simulink model "SystemComposerModel"  (R2022b)
settings: Solver=VariableStepAuto  StartTime=0.0  StopTime=10.0  RelTol=1e-3
(part 1 of 3)
settings Model: Creator=Daniel Sotelo  LastModifiedBy=teres
settings DebuggingCC: UnconnectedInputMsg=warning  UnconnectedOutputMsg=warning  UnconnectedLineMsg=warning
settings ModelReferenceCC: EnableRefExpFcnMdlSchedulingChecks=on
settings RTWCC: DLArmComputeVersion=19.05

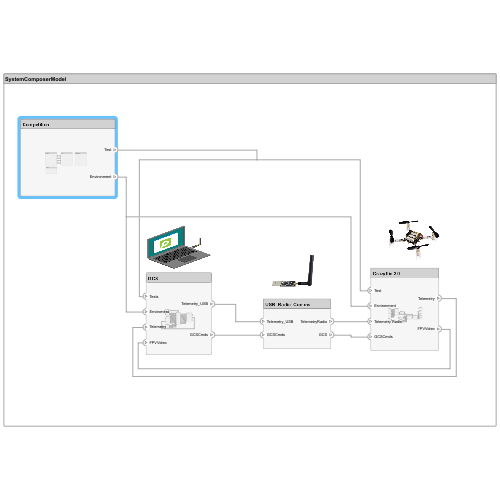
[thumbnail: Simulink's stored preview of the top-level diagram]
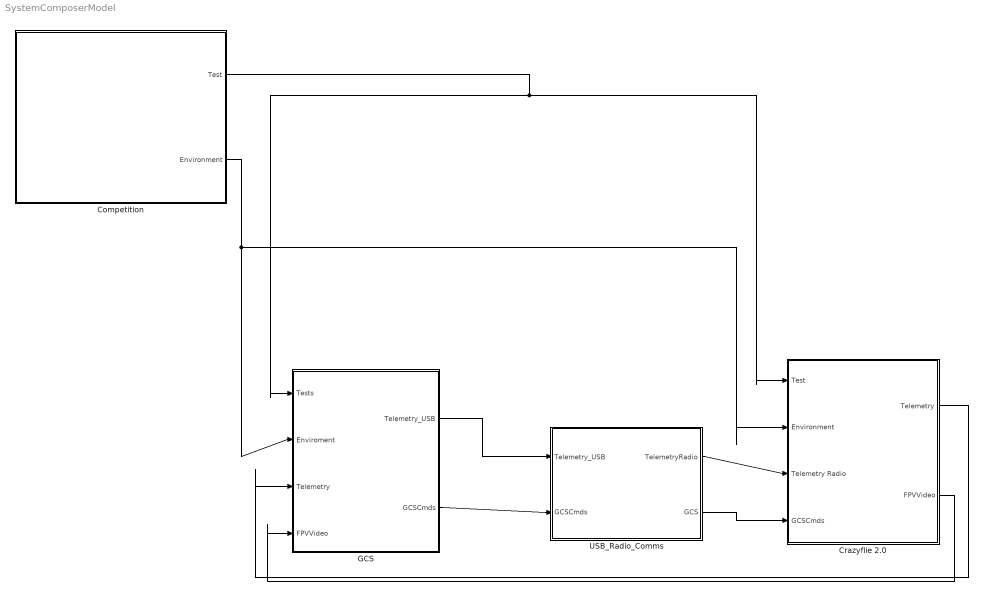
== system SystemComposerModel ==
  Competition : Subsystem
      settings: PortSchema="{\"entries\":[{\"content\":{\"headerSize\":26,\"margin\":15,\"minimumSpacing\":25,\"sides\":[{\"content\":{\"connectorIds\":[]},\"type\":\"ConnectorPlacement.EquallySpacedRectSide\",\"uuid\":\"fc8f1965-bed8-4a6e-9b63-950a000149c8\"},{\"content\":{\"connectorIds\":[\"Out1\",\"Out2\"],\"side\":\"RIGHT\"},\"type\":\"ConnectorPlacement.EquallySpacedRectSide\",\"uuid\":\"2c9d1f86-4f7d-4bcb-a56b-8c273be091e3\"},{\"content\":{\"connectorIds\":[],\"side\":\"TOP\"},\"type\":\"ConnectorPlacement.EquallySpacedRectSide\",\"uuid\":\"bf2fc06d-f400-4269-8d37-da038df58cba\"}]},\"type\":\"ConnectorPlacement.EquallySpacedConnector\",\"uuid\":\"4137853d-6a53-4ff1-a45c-0a11cac79d77\"}],\"packageUris\":[\"http://schema.mathworks.com/mf0/Connector/R2020b\"],\"version\":\"1.0\"}"
  Crazyflie 2.0 : Subsystem
      settings: PortSchema="{\"entries\":[{\"content\":{\"headerSize\":26,\"margin\":15,\"minimumSpacing\":25,\"sides\":[{\"content\":{\"connectorIds\":[\"In1\",\"In2\",\"In3\",\"In4\"]},\"type\":\"ConnectorPlacement.EquallySpacedRectSide\",\"uuid\":\"85361f62-a72a-43f7-8205-2bd06b4635eb\"},{\"content\":{\"connectorIds\":[\"Out1\",\"Out2\"],\"side\":\"RIGHT\"},\"type\":\"ConnectorPlacement.EquallySpacedRectSide\",\"uuid\":\"785bca03-4c5c-4ff5-9bb5-891ad5972055\"},{\"content\":{\"connectorIds\":[],\"side\":\"TOP\"},\"type\":\"ConnectorPlacement.EquallySpacedRectSide\",\"uuid\":\"4b8cfef5-38ba-456f-a828-b5cb7f165aef\"}]},\"type\":\"ConnectorPlacement.EquallySpacedConnector\",\"uuid\":\"8dffc657-0173-4421-b98e-59d56a4d09a6\"}],\"packageUris\":[\"http://schema.mathworks.com/mf0/Connector/R2020b\"],\"version\":\"1.0\"}"
  GCS : Subsystem
      settings: PortSchema="{\"entries\":[{\"content\":{\"headerSize\":26,\"margin\":15,\"minimumSpacing\":25,\"sides\":[{\"content\":{\"connectorIds\":[\"In1\",\"In2\",\"In3\",\"In4\"]},\"type\":\"ConnectorPlacement.EquallySpacedRectSide\",\"uuid\":\"b8d7d09c-e9ae-43de-8d46-f99ec2351e24\"},{\"content\":{\"connectorIds\":[\"Out1\",\"Out2\"],\"side\":\"RIGHT\"},\"type\":\"ConnectorPlacement.EquallySpacedRectSide\",\"uuid\":\"4693648e-b0a2-4db8-a983-4bee2f51d894\"},{\"content\":{\"connectorIds\":[],\"side\":\"TOP\"},\"type\":\"ConnectorPlacement.EquallySpacedRectSide\",\"uuid\":\"9f0e5fe3-4fa7-4597-a4df-94b2d5032736\"}]},\"type\":\"ConnectorPlacement.EquallySpacedConnector\",\"uuid\":\"297bf07a-4341-4423-8aed-0af6edbe7857\"}],\"packageUris\":[\"http://schema.mathworks.com/mf0/Connector/R2020b\"],\"version\":\"1.0\"}"
  USB_Radio_Comms : Subsystem
      settings: PortSchema="{\"entries\":[{\"content\":{\"headerSize\":26,\"margin\":15,\"minimumSpacing\":25,\"sides\":[{\"content\":{\"connectorIds\":[\"In1\",\"In2\"]},\"type\":\"ConnectorPlacement.EquallySpacedRectSide\",\"uuid\":\"3060b7dc-7094-4575-9bf7-25188df55435\"},{\"content\":{\"connectorIds\":[\"Out1\",\"Out2\"],\"side\":\"RIGHT\"},\"type\":\"ConnectorPlacement.EquallySpacedRectSide\",\"uuid\":\"b9a04f2f-3a87-4657-b996-549de6fa8c5c\"},{\"content\":{\"connectorIds\":[],\"side\":\"TOP\"},\"type\":\"ConnectorPlacement.EquallySpacedRectSide\",\"uuid\":\"d83a1232-3c8e-4ec4-b9bc-48e288d7909e\"}]},\"type\":\"ConnectorPlacement.EquallySpacedConnector\",\"uuid\":\"e5d04a2f-bf26-4a7e-a63c-4de52d3a604d\"}],\"packageUris\":[\"http://schema.mathworks.com/mf0/Connector/R2020b\"],\"version\":\"1.0\"}"
  wires:
  Crazyflie 2.0/1(Telemetry) -> GCS/3(Telemetry)
  Crazyflie 2.0/2(FPVVideo) -> GCS/4(FPVVideo)
  Competition/1(Test) -> GCS/1(Tests), Crazyflie 2.0/1(Test)
  Competition/2(Environment) -> Crazyflie 2.0/2(Environment), GCS/2(Enviroment)
  GCS/1(Telemetry_USB) -> USB_Radio_Comms/1(Telemetry_USB)
  GCS/2(GCSCmds) -> USB_Radio_Comms/2(GCSCmds)
  USB_Radio_Comms/1(TelemetryRadio) -> Crazyflie 2.0/3("Telemetry Radio ")
  USB_Radio_Comms/2(GCS) -> Crazyflie 2.0/4(GCSCmds)

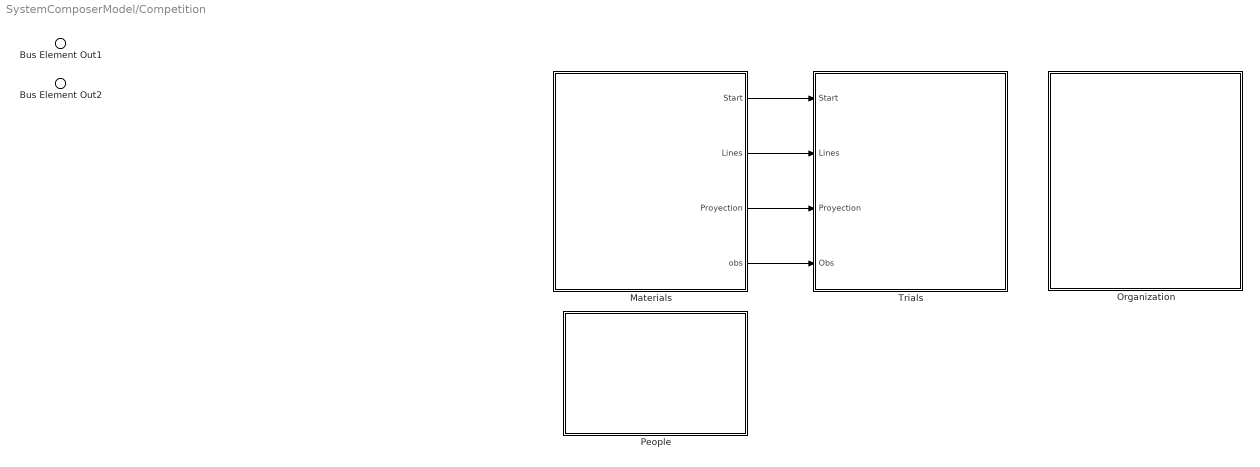
== system SystemComposerModel/Competition ==
  Materials : Subsystem
      settings: PortSchema="{\"entries\":[{\"content\":{\"headerSize\":26,\"margin\":15,\"minimumSpacing\":25,\"sides\":[{\"content\":{\"connectorIds\":[]},\"type\":\"ConnectorPlacement.EquallySpacedRectSide\",\"uuid\":\"036f86a6-46aa-44c7-aacf-5c5bf73f23a6\"},{\"content\":{\"connectorIds\":[\"Out1\",\"Out2\",\"Out3\",\"Out4\"],\"side\":\"RIGHT\"},\"type\":\"ConnectorPlacement.EquallySpacedRectSide\",\"uuid\":\"14d10c07-b9d4-4e69-9885-676f86520516\"},{\"content\":{\"connectorIds\":[],\"side\":\"TOP\"},\"type\":\"ConnectorPlacement.EquallySpacedRectSide\",\"uuid\":\"507b0a08-3f41-418e-b758-bf3c30bff976\"}]},\"type\":\"ConnectorPlacement.EquallySpacedConnector\",\"uuid\":\"3d035927-e5ab-4804-9878-aec4e1ed4314\"}],\"packageUris\":[\"http://schema.mathworks.com/mf0/Connector/R2020b\"],\"version\":\"1.0\"}"
  Organization : Subsystem
      settings: PortSchema="{\"entries\":[{\"content\":{\"headerSize\":26,\"margin\":15,\"minimumSpacing\":25,\"sides\":[{\"content\":{\"connectorIds\":[]},\"type\":\"ConnectorPlacement.EquallySpacedRectSide\",\"uuid\":\"036f86a6-46aa-44c7-aacf-5c5bf73f23a6\"},{\"content\":{\"connectorIds\":[],\"side\":\"RIGHT\"},\"type\":\"ConnectorPlacement.EquallySpacedRectSide\",\"uuid\":\"14d10c07-b9d4-4e69-9885-676f86520516\"},{\"content\":{\"connectorIds\":[],\"side\":\"TOP\"},\"type\":\"ConnectorPlacement.EquallySpacedRectSide\",\"uuid\":\"507b0a08-3f41-418e-b758-bf3c30bff976\"}]},\"type\":\"ConnectorPlacement.EquallySpacedConnector\",\"uuid\":\"3d035927-e5ab-4804-9878-aec4e1ed4314\"}],\"packageUris\":[\"http://schema.mathworks.com/mf0/Connector/R2020b\"],\"version\":\"1.0\"}"
  People : Subsystem
      settings: PortSchema="{\"entries\":[{\"content\":{\"headerSize\":26,\"margin\":15,\"minimumSpacing\":25,\"sides\":[{\"content\":{\"connectorIds\":[]},\"type\":\"ConnectorPlacement.EquallySpacedRectSide\",\"uuid\":\"036f86a6-46aa-44c7-aacf-5c5bf73f23a6\"},{\"content\":{\"connectorIds\":[],\"side\":\"RIGHT\"},\"type\":\"ConnectorPlacement.EquallySpacedRectSide\",\"uuid\":\"14d10c07-b9d4-4e69-9885-676f86520516\"},{\"content\":{\"connectorIds\":[],\"side\":\"TOP\"},\"type\":\"ConnectorPlacement.EquallySpacedRectSide\",\"uuid\":\"507b0a08-3f41-418e-b758-bf3c30bff976\"}]},\"type\":\"ConnectorPlacement.EquallySpacedConnector\",\"uuid\":\"3d035927-e5ab-4804-9878-aec4e1ed4314\"}],\"packageUris\":[\"http://schema.mathworks.com/mf0/Connector/R2020b\"],\"version\":\"1.0\"}"
  Trials : Subsystem
      settings: PortSchema="{\"entries\":[{\"content\":{\"headerSize\":26,\"margin\":15,\"minimumSpacing\":25,\"sides\":[{\"content\":{\"connectorIds\":[\"In1\",\"In2\",\"In3\",\"In4\"]},\"type\":\"ConnectorPlacement.EquallySpacedRectSide\",\"uuid\":\"036f86a6-46aa-44c7-aacf-5c5bf73f23a6\"},{\"content\":{\"connectorIds\":[],\"side\":\"RIGHT\"},\"type\":\"ConnectorPlacement.EquallySpacedRectSide\",\"uuid\":\"14d10c07-b9d4-4e69-9885-676f86520516\"},{\"content\":{\"connectorIds\":[],\"side\":\"TOP\"},\"type\":\"ConnectorPlacement.EquallySpacedRectSide\",\"uuid\":\"507b0a08-3f41-418e-b758-bf3c30bff976\"}]},\"type\":\"ConnectorPlacement.EquallySpacedConnector\",\"uuid\":\"3d035927-e5ab-4804-9878-aec4e1ed4314\"}],\"packageUris\":[\"http://schema.mathworks.com/mf0/Connector/R2020b\"],\"version\":\"1.0\"}"
  Bus Element Out1 : Outport  PortName=Test
  Bus Element Out2 : Outport  Port=2  PortName=Environment
  wires:
  Materials/2(Lines) -> Trials/2(Lines)
  Materials/3(Proyection) -> Trials/3(Proyection)
  Materials/4(obs) -> Trials/4(Obs)
  Materials/1(Start) -> Trials/1(Start)

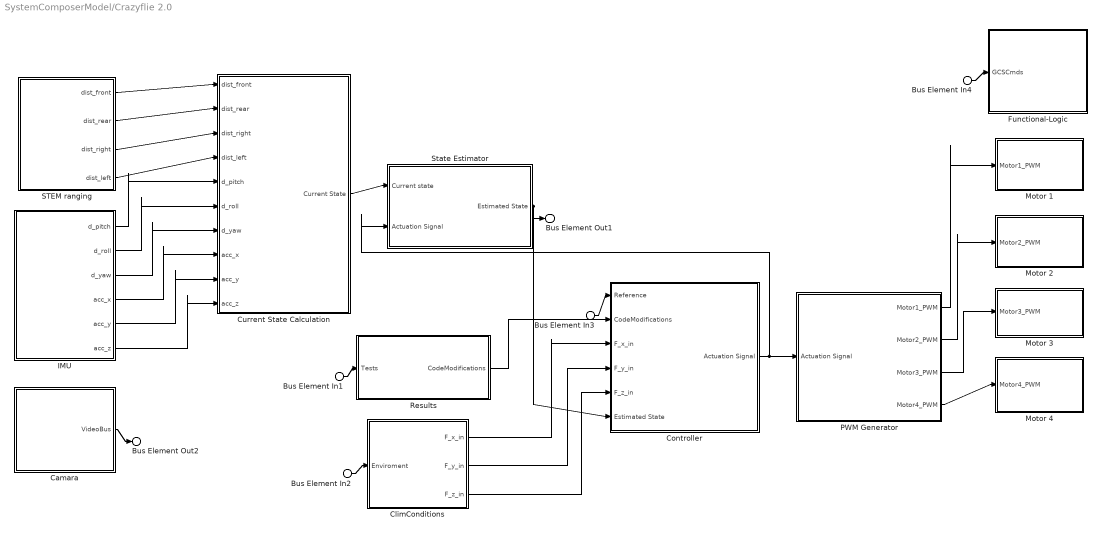
== system SystemComposerModel/Crazyflie 2.0 ==
  Bus Element In1 : Inport  PortName=Test
  Bus Element In2 : Inport  Port=2  PortName=Environment
  Bus Element In3 : Inport  Port=3  PortName=Telemetry Radio
  Bus Element In4 : Inport  Port=4  PortName=GCSCmds
  Camara : Subsystem
      settings: PortSchema="{\"entries\":[{\"content\":{\"headerSize\":26,\"margin\":15,\"minimumSpacing\":25,\"sides\":[{\"content\":{\"connectorIds\":[]},\"type\":\"ConnectorPlacement.EquallySpacedRectSide\",\"uuid\":\"85361f62-a72a-43f7-8205-2bd06b4635eb\"},{\"content\":{\"connectorIds\":[\"Out1\"],\"side\":\"RIGHT\"},\"type\":\"ConnectorPlacement.EquallySpacedRectSide\",\"uuid\":\"785bca03-4c5c-4ff5-9bb5-891ad5972055\"},{\"content\":{\"connectorIds\":[],\"side\":\"TOP\"},\"type\":\"ConnectorPlacement.EquallySpacedRectSide\",\"uuid\":\"4b8cfef5-38ba-456f-a828-b5cb7f165aef\"}]},\"type\":\"ConnectorPlacement.EquallySpacedConnector\",\"uuid\":\"8dffc657-0173-4421-b98e-59d56a4d09a6\"}],\"packageUris\":[\"http://schema.mathworks.com/mf0/Connector/R2020b\"],\"version\":\"1.0\"}"
  ClimConditions : Subsystem
      settings: PortSchema="{\"entries\":[{\"content\":{\"headerSize\":26,\"margin\":15,\"minimumSpacing\":25,\"sides\":[{\"content\":{\"connectorIds\":[\"In1\"]},\"type\":\"ConnectorPlacement.EquallySpacedRectSide\",\"uuid\":\"b8d7d09c-e9ae-43de-8d46-f99ec2351e24\"},{\"content\":{\"connectorIds\":[\"Out1\",\"Out2\",\"Out3\"],\"side\":\"RIGHT\"},\"type\":\"ConnectorPlacement.EquallySpacedRectSide\",\"uuid\":\"4693648e-b0a2-4db8-a983-4bee2f51d894\"},{\"content\":{\"connectorIds\":[],\"side\":\"TOP\"},\"type\":\"ConnectorPlacement.EquallySpacedRectSide\",\"uuid\":\"9f0e5fe3-4fa7-4597-a4df-94b2d5032736\"}]},\"type\":\"ConnectorPlacement.EquallySpacedConnector\",\"uuid\":\"297bf07a-4341-4423-8aed-0af6edbe7857\"}],\"packageUris\":[\"http://schema.mathworks.com/mf0/Connector/R2020b\"],\"version\":\"1.0\"}"
  Controller : Subsystem
      settings: PortSchema="{\"entries\":[{\"content\":{\"headerSize\":26,\"margin\":15,\"minimumSpacing\":25,\"sides\":[{\"content\":{\"connectorIds\":[\"In1\",\"In2\",\"In3\",\"In4\",\"In5\",\"In6\"]},\"type\":\"ConnectorPlacement.EquallySpacedRectSide\",\"uuid\":\"05353883-9549-4dc8-9a1c-5d1ae12c1484\"},{\"content\":{\"connectorIds\":[\"Out1\"],\"side\":\"RIGHT\"},\"type\":\"ConnectorPlacement.EquallySpacedRectSide\",\"uuid\":\"006c1520-45b5-4971-bef2-ea03737e2b23\"},{\"content\":{\"connectorIds\":[],\"side\":\"TOP\"},\"type\":\"ConnectorPlacement.EquallySpacedRectSide\",\"uuid\":\"e61f6cee-2c78-4df2-8cd1-114268c994e4\"}]},\"type\":\"ConnectorPlacement.EquallySpacedConnector\",\"uuid\":\"e2af53a5-fa78-4528-a754-d30d2cd5caf8\"}],\"packageUris\":[\"http://schema.mathworks.com/mf0/Connector/R2020b\"],\"version\":\"1.0\"}"
  Current State Calculation : Subsystem
      settings: PortSchema="{\"entries\":[{\"content\":{\"headerSize\":26,\"margin\":15,\"minimumSpacing\":25,\"sides\":[{\"content\":{\"connectorIds\":[\"In3\",\"In2\",\"In5\",\"In4\",\"In6\",\"In1\",\"In7\",\"In8\",\"In9\",\"In10\"]},\"type\":\"ConnectorPlacement.EquallySpacedRectSide\",\"uuid\":\"85361f62-a72a-43f7-8205-2bd06b4635eb\"},{\"content\":{\"connectorIds\":[\"Out1\"],\"side\":\"RIGHT\"},\"type\":\"ConnectorPlacement.EquallySpacedRectSide\",\"uuid\":\"785bca03-4c5c-4ff5-9bb5-891ad5972055\"},{\"content\":{\"connectorIds\":[],\"side\":\"TOP\"},\"type\":\"ConnectorPlacement.EquallySpacedRectSide\",\"uuid\":\"4b8cfef5-38ba-456f-a828-b5cb7f165aef\"},{\"content\":{\"connectorIds\":[],\"side\":\"BOTTOM\"},\"type\":\"ConnectorPlacement.EquallySpacedRectSide\",\"uuid\":\"ba702fc0-1fe6-457d-9dcb-728a63d76caf\"}]},\"type\":\"ConnectorPlacement.EquallySpacedConnector\",\"uuid\":\"8dffc657-0173-4421-b98e-59d56a4d09a6\"}],\"packageUris\":[\"http://schema.mathworks.com/mf0/Connector/R2020b\"],\"version\":\"1.0\"}"
  Functional-Logic : Subsystem
      settings: PortSchema="{\"entries\":[{\"content\":{\"headerSize\":26,\"margin\":15,\"minimumSpacing\":25,\"sides\":[{\"content\":{\"connectorIds\":[\"In1\"]},\"type\":\"ConnectorPlacement.EquallySpacedRectSide\",\"uuid\":\"85361f62-a72a-43f7-8205-2bd06b4635eb\"},{\"content\":{\"connectorIds\":[],\"side\":\"RIGHT\"},\"type\":\"ConnectorPlacement.EquallySpacedRectSide\",\"uuid\":\"785bca03-4c5c-4ff5-9bb5-891ad5972055\"},{\"content\":{\"connectorIds\":[],\"side\":\"TOP\"},\"type\":\"ConnectorPlacement.EquallySpacedRectSide\",\"uuid\":\"4b8cfef5-38ba-456f-a828-b5cb7f165aef\"}]},\"type\":\"ConnectorPlacement.EquallySpacedConnector\",\"uuid\":\"8dffc657-0173-4421-b98e-59d56a4d09a6\"}],\"packageUris\":[\"http://schema.mathworks.com/mf0/Connector/R2020b\"],\"version\":\"1.0\"}"
  IMU : Subsystem
      settings: PortSchema="{\"entries\":[{\"content\":{\"headerSize\":26,\"margin\":15,\"minimumSpacing\":25,\"sides\":[{\"content\":{\"connectorIds\":[]},\"type\":\"ConnectorPlacement.EquallySpacedRectSide\",\"uuid\":\"85361f62-a72a-43f7-8205-2bd06b4635eb\"},{\"content\":{\"connectorIds\":[\"Out1\",\"Out2\",\"Out3\",\"Out4\",\"Out5\",\"Out6\"],\"side\":\"RIGHT\"},\"type\":\"ConnectorPlacement.EquallySpacedRectSide\",\"uuid\":\"785bca03-4c5c-4ff5-9bb5-891ad5972055\"},{\"content\":{\"connectorIds\":[],\"side\":\"TOP\"},\"type\":\"ConnectorPlacement.EquallySpacedRectSide\",\"uuid\":\"4b8cfef5-38ba-456f-a828-b5cb7f165aef\"}]},\"type\":\"ConnectorPlacement.EquallySpacedConnector\",\"uuid\":\"8dffc657-0173-4421-b98e-59d56a4d09a6\"}],\"packageUris\":[\"http://schema.mathworks.com/mf0/Connector/R2020b\"],\"version\":\"1.0\"}"
  Motor 1 : Subsystem
      settings: PortSchema="{\"entries\":[{\"content\":{\"headerSize\":26,\"margin\":15,\"minimumSpacing\":25,\"sides\":[{\"content\":{\"connectorIds\":[\"In1\"]},\"type\":\"ConnectorPlacement.EquallySpacedRectSide\",\"uuid\":\"05353883-9549-4dc8-9a1c-5d1ae12c1484\"},{\"content\":{\"connectorIds\":[],\"side\":\"RIGHT\"},\"type\":\"ConnectorPlacement.EquallySpacedRectSide\",\"uuid\":\"006c1520-45b5-4971-bef2-ea03737e2b23\"},{\"content\":{\"connectorIds\":[],\"side\":\"TOP\"},\"type\":\"ConnectorPlacement.EquallySpacedRectSide\",\"uuid\":\"e61f6cee-2c78-4df2-8cd1-114268c994e4\"}]},\"type\":\"ConnectorPlacement.EquallySpacedConnector\",\"uuid\":\"e2af53a5-fa78-4528-a754-d30d2cd5caf8\"}],\"packageUris\":[\"http://schema.mathworks.com/mf0/Connector/R2020b\"],\"version\":\"1.0\"}"
  Motor 2 : Subsystem
      settings: PortSchema="{\"entries\":[{\"content\":{\"headerSize\":26,\"margin\":15,\"minimumSpacing\":25,\"sides\":[{\"content\":{\"connectorIds\":[\"In1\"]},\"type\":\"ConnectorPlacement.EquallySpacedRectSide\",\"uuid\":\"05353883-9549-4dc8-9a1c-5d1ae12c1484\"},{\"content\":{\"connectorIds\":[],\"side\":\"RIGHT\"},\"type\":\"ConnectorPlacement.EquallySpacedRectSide\",\"uuid\":\"006c1520-45b5-4971-bef2-ea03737e2b23\"},{\"content\":{\"connectorIds\":[],\"side\":\"TOP\"},\"type\":\"ConnectorPlacement.EquallySpacedRectSide\",\"uuid\":\"e61f6cee-2c78-4df2-8cd1-114268c994e4\"}]},\"type\":\"ConnectorPlacement.EquallySpacedConnector\",\"uuid\":\"e2af53a5-fa78-4528-a754-d30d2cd5caf8\"}],\"packageUris\":[\"http://schema.mathworks.com/mf0/Connector/R2020b\"],\"version\":\"1.0\"}"
  Motor 3 : Subsystem
      settings: PortSchema="{\"entries\":[{\"content\":{\"headerSize\":26,\"margin\":15,\"minimumSpacing\":25,\"sides\":[{\"content\":{\"connectorIds\":[\"In1\"]},\"type\":\"ConnectorPlacement.EquallySpacedRectSide\",\"uuid\":\"05353883-9549-4dc8-9a1c-5d1ae12c1484\"},{\"content\":{\"connectorIds\":[],\"side\":\"RIGHT\"},\"type\":\"ConnectorPlacement.EquallySpacedRectSide\",\"uuid\":\"006c1520-45b5-4971-bef2-ea03737e2b23\"},{\"content\":{\"connectorIds\":[],\"side\":\"TOP\"},\"type\":\"ConnectorPlacement.EquallySpacedRectSide\",\"uuid\":\"e61f6cee-2c78-4df2-8cd1-114268c994e4\"}]},\"type\":\"ConnectorPlacement.EquallySpacedConnector\",\"uuid\":\"e2af53a5-fa78-4528-a754-d30d2cd5caf8\"}],\"packageUris\":[\"http://schema.mathworks.com/mf0/Connector/R2020b\"],\"version\":\"1.0\"}"
  Motor 4 : Subsystem
      settings: PortSchema="{\"entries\":[{\"content\":{\"headerSize\":26,\"margin\":15,\"minimumSpacing\":25,\"sides\":[{\"content\":{\"connectorIds\":[\"In1\"]},\"type\":\"ConnectorPlacement.EquallySpacedRectSide\",\"uuid\":\"05353883-9549-4dc8-9a1c-5d1ae12c1484\"},{\"content\":{\"connectorIds\":[],\"side\":\"RIGHT\"},\"type\":\"ConnectorPlacement.EquallySpacedRectSide\",\"uuid\":\"006c1520-45b5-4971-bef2-ea03737e2b23\"},{\"content\":{\"connectorIds\":[],\"side\":\"TOP\"},\"type\":\"ConnectorPlacement.EquallySpacedRectSide\",\"uuid\":\"e61f6cee-2c78-4df2-8cd1-114268c994e4\"}]},\"type\":\"ConnectorPlacement.EquallySpacedConnector\",\"uuid\":\"e2af53a5-fa78-4528-a754-d30d2cd5caf8\"}],\"packageUris\":[\"http://schema.mathworks.com/mf0/Connector/R2020b\"],\"version\":\"1.0\"}"
  PWM Generator : Subsystem
      settings: PortSchema="{\"entries\":[{\"content\":{\"headerSize\":26,\"margin\":15,\"minimumSpacing\":25,\"sides\":[{\"content\":{\"connectorIds\":[\"In1\"]},\"type\":\"ConnectorPlacement.EquallySpacedRectSide\",\"uuid\":\"05353883-9549-4dc8-9a1c-5d1ae12c1484\"},{\"content\":{\"connectorIds\":[\"Out1\",\"Out2\",\"Out3\",\"Out4\"],\"side\":\"RIGHT\"},\"type\":\"ConnectorPlacement.EquallySpacedRectSide\",\"uuid\":\"006c1520-45b5-4971-bef2-ea03737e2b23\"},{\"content\":{\"connectorIds\":[],\"side\":\"TOP\"},\"type\":\"ConnectorPlacement.EquallySpacedRectSide\",\"uuid\":\"e61f6cee-2c78-4df2-8cd1-114268c994e4\"}]},\"type\":\"ConnectorPlacement.EquallySpacedConnector\",\"uuid\":\"e2af53a5-fa78-4528-a754-d30d2cd5caf8\"}],\"packageUris\":[\"http://schema.mathworks.com/mf0/Connector/R2020b\"],\"version\":\"1.0\"}"
  Results : Subsystem
      settings: PortSchema="{\"entries\":[{\"content\":{\"headerSize\":26,\"margin\":15,\"minimumSpacing\":25,\"sides\":[{\"content\":{\"connectorIds\":[\"In1\"]},\"type\":\"ConnectorPlacement.EquallySpacedRectSide\",\"uuid\":\"b8d7d09c-e9ae-43de-8d46-f99ec2351e24\"},{\"content\":{\"connectorIds\":[\"Out1\"],\"side\":\"RIGHT\"},\"type\":\"ConnectorPlacement.EquallySpacedRectSide\",\"uuid\":\"4693648e-b0a2-4db8-a983-4bee2f51d894\"},{\"content\":{\"connectorIds\":[],\"side\":\"TOP\"},\"type\":\"ConnectorPlacement.EquallySpacedRectSide\",\"uuid\":\"9f0e5fe3-4fa7-4597-a4df-94b2d5032736\"}]},\"type\":\"ConnectorPlacement.EquallySpacedConnector\",\"uuid\":\"297bf07a-4341-4423-8aed-0af6edbe7857\"}],\"packageUris\":[\"http://schema.mathworks.com/mf0/Connector/R2020b\"],\"version\":\"1.0\"}"
  STEM ranging : Subsystem
      settings: PortSchema="{\"entries\":[{\"content\":{\"headerSize\":26,\"margin\":15,\"minimumSpacing\":25,\"sides\":[{\"content\":{\"connectorIds\":[]},\"type\":\"ConnectorPlacement.EquallySpacedRectSide\",\"uuid\":\"85361f62-a72a-43f7-8205-2bd06b4635eb\"},{\"content\":{\"connectorIds\":[\"Out1\",\"Out2\",\"Out3\",\"Out4\"],\"side\":\"RIGHT\"},\"type\":\"ConnectorPlacement.EquallySpacedRectSide\",\"uuid\":\"785bca03-4c5c-4ff5-9bb5-891ad5972055\"},{\"content\":{\"connectorIds\":[],\"side\":\"TOP\"},\"type\":\"ConnectorPlacement.EquallySpacedRectSide\",\"uuid\":\"4b8cfef5-38ba-456f-a828-b5cb7f165aef\"}]},\"type\":\"ConnectorPlacement.EquallySpacedConnector\",\"uuid\":\"8dffc657-0173-4421-b98e-59d56a4d09a6\"}],\"packageUris\":[\"http://schema.mathworks.com/mf0/Connector/R2020b\"],\"version\":\"1.0\"}"
  State Estimator : Subsystem
      settings: PortSchema="{\"entries\":[{\"content\":{\"headerSize\":26,\"margin\":15,\"minimumSpacing\":25,\"sides\":[{\"content\":{\"connectorIds\":[\"In1\",\"In2\"]},\"type\":\"ConnectorPlacement.EquallySpacedRectSide\",\"uuid\":\"05353883-9549-4dc8-9a1c-5d1ae12c1484\"},{\"content\":{\"connectorIds\":[\"Out1\"],\"side\":\"RIGHT\"},\"type\":\"ConnectorPlacement.EquallySpacedRectSide\",\"uuid\":\"006c1520-45b5-4971-bef2-ea03737e2b23\"},{\"content\":{\"connectorIds\":[],\"side\":\"TOP\"},\"type\":\"ConnectorPlacement.EquallySpacedRectSide\",\"uuid\":\"e61f6cee-2c78-4df2-8cd1-114268c994e4\"}]},\"type\":\"ConnectorPlacement.EquallySpacedConnector\",\"uuid\":\"e2af53a5-fa78-4528-a754-d30d2cd5caf8\"}],\"packageUris\":[\"http://schema.mathworks.com/mf0/Connector/R2020b\"],\"version\":\"1.0\"}"
  Bus Element Out1 : Outport  PortName=Telemetry
  Bus Element Out2 : Outport  Port=2  PortName=FPVVideo
  wires:
  PWM Generator/3(Motor3_PWM) -> Motor 3/1(Motor3_PWM)
  STEM ranging/1(dist_front) -> Current State Calculation/3(dist_front)
  ClimConditions/2(F_y_in) -> Controller/4(F_y_in)
  STEM ranging/2(dist_rear) -> Current State Calculation/2(dist_rear)
  IMU/4(acc_x) -> Current State Calculation/8(acc_x)
  STEM ranging/4(dist_left) -> Current State Calculation/4(dist_left)
  STEM ranging/3(dist_right) -> Current State Calculation/5(dist_right)
  IMU/3(d_yaw) -> Current State Calculation/7(d_yaw)
  Results/1(CodeModifications) -> Controller/2(CodeModifications)
  IMU/2(d_roll) -> Current State Calculation/1(d_roll)
  IMU/1(d_pitch) -> Current State Calculation/6(d_pitch)
  IMU/5(acc_y) -> Current State Calculation/9(acc_y)
  IMU/6(acc_z) -> Current State Calculation/10(acc_z)
  Bus Element In4/1 -> Functional-Logic/1(GCSCmds)
  Camara/1(VideoBus) -> Bus Element Out2/1
  Current State Calculation/1(Current State) -> State Estimator/1(Current state)
  PWM Generator/2(Motor2_PWM) -> Motor 2/1(Motor2_PWM)
  Bus Element In2/1 -> ClimConditions/1(Enviroment)
  Bus Element In1/1 -> Results/1(Tests)
  PWM Generator/4(Motor4_PWM) -> Motor 4/1(Motor4_PWM)
  State Estimator/1(Estimated State) -> Controller/6(Estimated State), Bus Element Out1/1
  Controller/1(Actuation Signal) -> PWM Generator/1(Actuation Signal), State Estimator/2(Actuation Signal)
  Bus Element In3/1 -> Controller/1(Reference)
  ClimConditions/3(F_z_in) -> Controller/5(F_z_in)
  ClimConditions/1(F_x_in) -> Controller/3(F_x_in)
  PWM Generator/1(Motor1_PWM) -> Motor 1/1(Motor1_PWM)

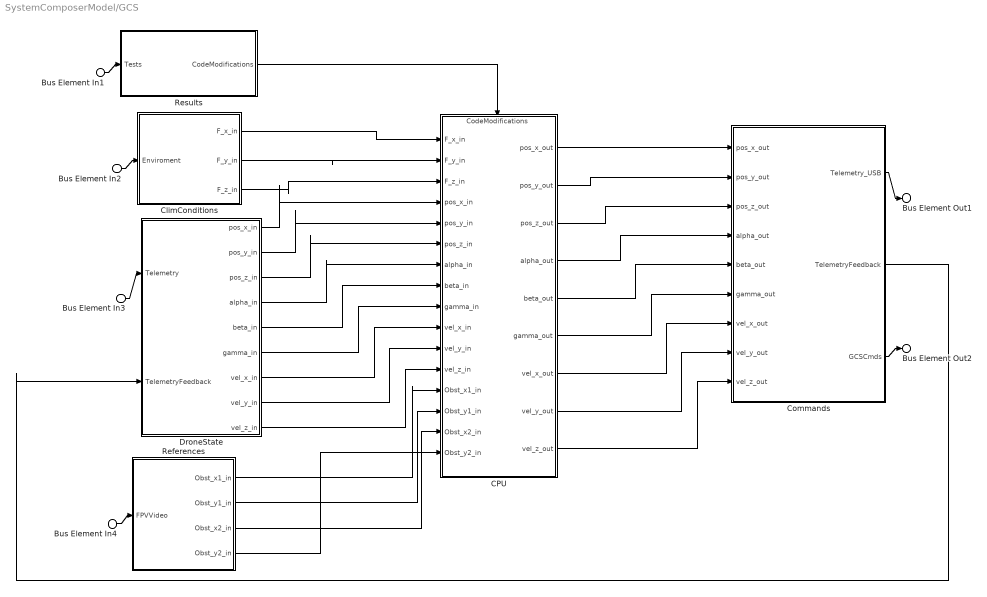
== system SystemComposerModel/GCS ==
  Bus Element In1 : Inport  PortName=Tests
  Bus Element In2 : Inport  Port=2  PortName=Enviroment
  Bus Element In3 : Inport  Port=3  PortName=Telemetry
  Bus Element In4 : Inport  Port=4  PortName=FPVVideo
  CPU : Subsystem
      settings: PortSchema="{\"entries\":[{\"content\":{\"headerSize\":26,\"margin\":15,\"minimumSpacing\":25,\"sides\":[{\"content\":{\"connectorIds\":[\"In2\",\"In3\",\"In4\",\"In5\",\"In6\",\"In7\",\"In8\",\"In9\",\"In10\",\"In11\",\"In12\",\"In13\",\"In14\",\"In15\",\"In16\",\"In17\"]},\"type\":\"ConnectorPlacement.EquallySpacedRectSide\",\"uuid\":\"b8d7d09c-e9ae-43de-8d46-f99ec2351e24\"},{\"content\":{\"connectorIds\":[\"Out1\",\"Out2\",\"Out3\",\"Out4\",\"Out5\",\"Out6\",\"Out7\",\"Out8\",\"Out9\"],\"side\":\"RIGHT\"},\"type\":\"ConnectorPlacement.EquallySpacedRectSide\",\"uuid\":\"4693648e-b0a2-4db8-a983-4bee2f51d894\"},{\"content\":{\"connectorIds\":[\"In1\"],\"side\":\"TOP\"},\"type\":\"ConnectorPlacement.EquallySpacedRectSide\",\"uuid\":\"9f0e5fe3-4fa7-4597-a4df-94b2d5032736\"}]},\"type\":\"ConnectorPlacement.EquallySpacedConnector\",\"uuid\":\"297bf07a-4341-4423-8aed-0af6edbe7857\"}],\"packageUris\":[\"http://schema.mathworks.com/mf0/Connector/R2020b\"],\"version\":\"1.0\"}"
  ClimConditions : Subsystem
      settings: PortSchema="{\"entries\":[{\"content\":{\"headerSize\":26,\"margin\":15,\"minimumSpacing\":25,\"sides\":[{\"content\":{\"connectorIds\":[\"In1\"]},\"type\":\"ConnectorPlacement.EquallySpacedRectSide\",\"uuid\":\"b8d7d09c-e9ae-43de-8d46-f99ec2351e24\"},{\"content\":{\"connectorIds\":[\"Out1\",\"Out2\",\"Out3\"],\"side\":\"RIGHT\"},\"type\":\"ConnectorPlacement.EquallySpacedRectSide\",\"uuid\":\"4693648e-b0a2-4db8-a983-4bee2f51d894\"},{\"content\":{\"connectorIds\":[],\"side\":\"TOP\"},\"type\":\"ConnectorPlacement.EquallySpacedRectSide\",\"uuid\":\"9f0e5fe3-4fa7-4597-a4df-94b2d5032736\"}]},\"type\":\"ConnectorPlacement.EquallySpacedConnector\",\"uuid\":\"297bf07a-4341-4423-8aed-0af6edbe7857\"}],\"packageUris\":[\"http://schema.mathworks.com/mf0/Connector/R2020b\"],\"version\":\"1.0\"}"
  Commands : Subsystem
      settings: PortSchema="{\"entries\":[{\"content\":{\"headerSize\":26,\"margin\":15,\"minimumSpacing\":25,\"sides\":[{\"content\":{\"connectorIds\":[\"In1\",\"In2\",\"In3\",\"In4\",\"In5\",\"In6\",\"In7\",\"In8\",\"In9\"]},\"type\":\"ConnectorPlacement.EquallySpacedRectSide\",\"uuid\":\"b8d7d09c-e9ae-43de-8d46-f99ec2351e24\"},{\"content\":{\"connectorIds\":[\"Out1\",\"Out2\",\"Out3\"],\"side\":\"RIGHT\"},\"type\":\"ConnectorPlacement.EquallySpacedRectSide\",\"uuid\":\"4693648e-b0a2-4db8-a983-4bee2f51d894\"},{\"content\":{\"connectorIds\":[],\"side\":\"TOP\"},\"type\":\"ConnectorPlacement.EquallySpacedRectSide\",\"uuid\":\"9f0e5fe3-4fa7-4597-a4df-94b2d5032736\"}]},\"type\":\"ConnectorPlacement.EquallySpacedConnector\",\"uuid\":\"297bf07a-4341-4423-8aed-0af6edbe7857\"}],\"packageUris\":[\"http://schema.mathworks.com/mf0/Connector/R2020b\"],\"version\":\"1.0\"}"
  DroneState : Subsystem
      settings: PortSchema="{\"entries\":[{\"content\":{\"headerSize\":26,\"margin\":15,\"minimumSpacing\":25,\"sides\":[{\"content\":{\"connectorIds\":[\"In1\",\"In2\"]},\"type\":\"ConnectorPlacement.EquallySpacedRectSide\",\"uuid\":\"b8d7d09c-e9ae-43de-8d46-f99ec2351e24\"},{\"content\":{\"connectorIds\":[\"Out1\",\"Out2\",\"Out3\",\"Out4\",\"Out5\",\"Out6\",\"Out7\",\"Out8\",\"Out9\"],\"side\":\"RIGHT\"},\"type\":\"ConnectorPlacement.EquallySpacedRectSide\",\"uuid\":\"4693648e-b0a2-4db8-a983-4bee2f51d894\"},{\"content\":{\"connectorIds\":[],\"side\":\"TOP\"},\"type\":\"ConnectorPlacement.EquallySpacedRectSide\",\"uuid\":\"9f0e5fe3-4fa7-4597-a4df-94b2d5032736\"}]},\"type\":\"ConnectorPlacement.EquallySpacedConnector\",\"uuid\":\"297bf07a-4341-4423-8aed-0af6edbe7857\"}],\"packageUris\":[\"http://schema.mathworks.com/mf0/Connector/R2020b\"],\"version\":\"1.0\"}"
  References : Subsystem
      settings: PortSchema="{\"entries\":[{\"content\":{\"headerSize\":26,\"margin\":15,\"minimumSpacing\":25,\"sides\":[{\"content\":{\"connectorIds\":[\"In1\"]},\"type\":\"ConnectorPlacement.EquallySpacedRectSide\",\"uuid\":\"b8d7d09c-e9ae-43de-8d46-f99ec2351e24\"},{\"content\":{\"connectorIds\":[\"Out1\",\"Out2\",\"Out3\",\"Out4\"],\"side\":\"RIGHT\"},\"type\":\"ConnectorPlacement.EquallySpacedRectSide\",\"uuid\":\"4693648e-b0a2-4db8-a983-4bee2f51d894\"},{\"content\":{\"connectorIds\":[],\"side\":\"TOP\"},\"type\":\"ConnectorPlacement.EquallySpacedRectSide\",\"uuid\":\"9f0e5fe3-4fa7-4597-a4df-94b2d5032736\"}]},\"type\":\"ConnectorPlacement.EquallySpacedConnector\",\"uuid\":\"297bf07a-4341-4423-8aed-0af6edbe7857\"}],\"packageUris\":[\"http://schema.mathworks.com/mf0/Connector/R2020b\"],\"version\":\"1.0\"}"
  Results : Subsystem
      settings: PortSchema="{\"entries\":[{\"content\":{\"headerSize\":26,\"margin\":15,\"minimumSpacing\":25,\"sides\":[{\"content\":{\"connectorIds\":[\"In1\"]},\"type\":\"ConnectorPlacement.EquallySpacedRectSide\",\"uuid\":\"b8d7d09c-e9ae-43de-8d46-f99ec2351e24\"},{\"content\":{\"connectorIds\":[\"Out1\"],\"side\":\"RIGHT\"},\"type\":\"ConnectorPlacement.EquallySpacedRectSide\",\"uuid\":\"4693648e-b0a2-4db8-a983-4bee2f51d894\"},{\"content\":{\"connectorIds\":[],\"side\":\"TOP\"},\"type\":\"ConnectorPlacement.EquallySpacedRectSide\",\"uuid\":\"9f0e5fe3-4fa7-4597-a4df-94b2d5032736\"}]},\"type\":\"ConnectorPlacement.EquallySpacedConnector\",\"uuid\":\"297bf07a-4341-4423-8aed-0af6edbe7857\"}],\"packageUris\":[\"http://schema.mathworks.com/mf0/Connector/R2020b\"],\"version\":\"1.0\"}"
  Bus Element Out1 : Outport  PortName=Telemetry_USB
  Bus Element Out2 : Outport  Port=2  PortName=GCSCmds
  wires:
  Bus Element In3/1 -> DroneState/1(Telemetry)
  Bus Element In4/1 -> References/1(FPVVideo)
  DroneState/1(pos_x_in) -> CPU/5(pos_x_in)
  DroneState/2(pos_y_in) -> CPU/6(pos_y_in)
  DroneState/3(pos_z_in) -> CPU/7(pos_z_in)
  DroneState/4(alpha_in) -> CPU/8(alpha_in)
  DroneState/5(beta_in) -> CPU/9(beta_in)
  DroneState/6(gamma_in) -> CPU/10(gamma_in)
  DroneState/7(vel_x_in) -> CPU/11(vel_x_in)
  DroneState/8(vel_y_in) -> CPU/12(vel_y_in)
  DroneState/9(vel_z_in) -> CPU/13(vel_z_in)
  References/1(Obst_x1_in) -> CPU/14(Obst_x1_in)
  References/2(Obst_y1_in) -> CPU/15(Obst_y1_in)
  References/3(Obst_x2_in) -> CPU/16(Obst_x2_in)
  References/4(Obst_y2_in) -> CPU/17(Obst_y2_in)
  Bus Element In2/1 -> ClimConditions/1(Enviroment)
  Bus Element In1/1 -> Results/1(Tests)
  ClimConditions/1(F_x_in) -> CPU/2(F_x_in)
  ClimConditions/2(F_y_in) -> CPU/3(F_y_in)
  ClimConditions/3(F_z_in) -> CPU/4(F_z_in)
  Results/1(CodeModifications) -> CPU/1(CodeModifications)
  CPU/1(pos_x_out) -> Commands/1(pos_x_out)
  CPU/2(pos_y_out) -> Commands/2(pos_y_out)
  CPU/3(pos_z_out) -> Commands/3(pos_z_out)
  CPU/4(alpha_out) -> Commands/4(alpha_out)
  CPU/5(beta_out) -> Commands/5(beta_out)
  CPU/6(gamma_out) -> Commands/6(gamma_out)
  CPU/7(vel_x_out) -> Commands/7(vel_x_out)
  CPU/8(vel_y_out) -> Commands/8(vel_y_out)
  CPU/9(vel_z_out) -> Commands/9(vel_z_out)
  Commands/3(GCSCmds) -> Bus Element Out2/1
  Commands/1(Telemetry_USB) -> Bus Element Out1/1
  Commands/2(TelemetryFeedback) -> DroneState/2(TelemetryFeedback)

== system SystemComposerModel/USB_Radio_Comms ==
  Bus Element In1 : Inport  PortName=Telemetry_USB
  Bus Element In2 : Inport  Port=2  PortName=GCSCmds
  Bus Element Out1 : Outport  PortName=TelemetryRadio
  Bus Element Out2 : Outport  Port=2  PortName=GCS

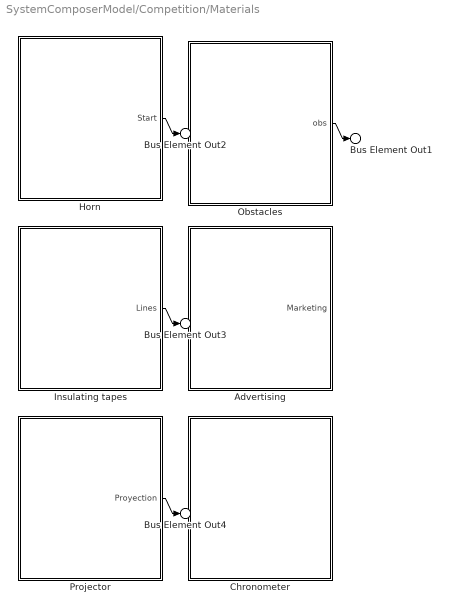
== system SystemComposerModel/Competition/Materials ==
  Advertising : Subsystem
      settings: PortSchema="{\"entries\":[{\"content\":{\"headerSize\":26,\"margin\":15,\"minimumSpacing\":25,\"sides\":[{\"content\":{\"connectorIds\":[]},\"type\":\"ConnectorPlacement.EquallySpacedRectSide\",\"uuid\":\"036f86a6-46aa-44c7-aacf-5c5bf73f23a6\"},{\"content\":{\"connectorIds\":[\"Out1\"],\"side\":\"RIGHT\"},\"type\":\"ConnectorPlacement.EquallySpacedRectSide\",\"uuid\":\"14d10c07-b9d4-4e69-9885-676f86520516\"},{\"content\":{\"connectorIds\":[],\"side\":\"TOP\"},\"type\":\"ConnectorPlacement.EquallySpacedRectSide\",\"uuid\":\"507b0a08-3f41-418e-b758-bf3c30bff976\"}]},\"type\":\"ConnectorPlacement.EquallySpacedConnector\",\"uuid\":\"3d035927-e5ab-4804-9878-aec4e1ed4314\"}],\"packageUris\":[\"http://schema.mathworks.com/mf0/Connector/R2020b\"],\"version\":\"1.0\"}"
  Chronometer : Subsystem  Description=|
      | Stopwatch needed to measure the time taken by the drone in the following tests:
      | 1. Speed test
      | 2. Tracking test
      | 3. Predefined obstacle test
      | 4. Random obstacle test
      | 5. Freestyle test
      | It will be sufficient to use the timer application included in the cell phones.
      settings: PortSchema="{\"entries\":[{\"content\":{\"headerSize\":26,\"margin\":15,\"minimumSpacing\":25,\"sides\":[{\"content\":{\"connectorIds\":[]},\"type\":\"ConnectorPlacement.EquallySpacedRectSide\",\"uuid\":\"036f86a6-46aa-44c7-aacf-5c5bf73f23a6\"},{\"content\":{\"connectorIds\":[],\"side\":\"RIGHT\"},\"type\":\"ConnectorPlacement.EquallySpacedRectSide\",\"uuid\":\"14d10c07-b9d4-4e69-9885-676f86520516\"},{\"content\":{\"connectorIds\":[],\"side\":\"TOP\"},\"type\":\"ConnectorPlacement.EquallySpacedRectSide\",\"uuid\":\"507b0a08-3f41-418e-b758-bf3c30bff976\"}]},\"type\":\"ConnectorPlacement.EquallySpacedConnector\",\"uuid\":\"3d035927-e5ab-4804-9878-aec4e1ed4314\"}],\"packageUris\":[\"http://schema.mathworks.com/mf0/Connector/R2020b\"],\"version\":\"1.0\"}"
  Horn : Subsystem  Description=|
      | Sound to mark the start of each test, in particular:
      | 1. Speed test
      | 2. Tracking test
      | 3. Predefined obstacle test
      | 4. Random obstacle test
      | 5. Freestyle test
      settings: PortSchema="{\"entries\":[{\"content\":{\"headerSize\":26,\"margin\":15,\"minimumSpacing\":25,\"sides\":[{\"content\":{\"connectorIds\":[]},\"type\":\"ConnectorPlacement.EquallySpacedRectSide\",\"uuid\":\"036f86a6-46aa-44c7-aacf-5c5bf73f23a6\"},{\"content\":{\"connectorIds\":[\"Out1\"],\"side\":\"RIGHT\"},\"type\":\"ConnectorPlacement.EquallySpacedRectSide\",\"uuid\":\"14d10c07-b9d4-4e69-9885-676f86520516\"},{\"content\":{\"connectorIds\":[],\"side\":\"TOP\"},\"type\":\"ConnectorPlacement.EquallySpacedRectSide\",\"uuid\":\"507b0a08-3f41-418e-b758-bf3c30bff976\"}]},\"type\":\"ConnectorPlacement.EquallySpacedConnector\",\"uuid\":\"3d035927-e5ab-4804-9878-aec4e1ed4314\"}],\"packageUris\":[\"http://schema.mathworks.com/mf0/Connector/R2020b\"],\"version\":\"1.0\"}"
  Insulating tapes : Subsystem  Description=|
      | Colored tape to delimit the course of each race, in particular:
      | 1. speed test: start and finish line (black) 
      | 2. Target test: marking on the ground the point from which the drone will take off (black).
      | 3. Trackline test: marking of the course (black color approx. 38mm thick, black color approx. 10mm thick, red color approx. 20mm thick), finish line (blue color).
      | 4. Predefined obstacle test: start and finish line.
      | 5. Random obstacle test: start and finish line.
      | 
      | For the above requirements, the following must be purchased:
      | 1 black tape approx. 38mm
      | 1 black tape approx. 10mm
      | 1 red tape approx. 20mm
      | 1 blue tape
      settings: PortSchema="{\"entries\":[{\"content\":{\"headerSize\":26,\"margin\":15,\"minimumSpacing\":25,\"sides\":[{\"content\":{\"connectorIds\":[]},\"type\":\"ConnectorPlacement.EquallySpacedRectSide\",\"uuid\":\"036f86a6-46aa-44c7-aacf-5c5bf73f23a6\"},{\"content\":{\"connectorIds\":[\"Out1\"],\"side\":\"RIGHT\"},\"type\":\"ConnectorPlacement.EquallySpacedRectSide\",\"uuid\":\"14d10c07-b9d4-4e69-9885-676f86520516\"},{\"content\":{\"connectorIds\":[],\"side\":\"TOP\"},\"type\":\"ConnectorPlacement.EquallySpacedRectSide\",\"uuid\":\"507b0a08-3f41-418e-b758-bf3c30bff976\"}]},\"type\":\"ConnectorPlacement.EquallySpacedConnector\",\"uuid\":\"3d035927-e5ab-4804-9878-aec4e1ed4314\"}],\"packageUris\":[\"http://schema.mathworks.com/mf0/Connector/R2020b\"],\"version\":\"1.0\"}"
  Obstacles : Subsystem
      settings: PortSchema="{\"entries\":[{\"content\":{\"headerSize\":26,\"margin\":15,\"minimumSpacing\":25,\"sides\":[{\"content\":{\"connectorIds\":[]},\"type\":\"ConnectorPlacement.EquallySpacedRectSide\",\"uuid\":\"036f86a6-46aa-44c7-aacf-5c5bf73f23a6\"},{\"content\":{\"connectorIds\":[\"Out1\"],\"side\":\"RIGHT\"},\"type\":\"ConnectorPlacement.EquallySpacedRectSide\",\"uuid\":\"14d10c07-b9d4-4e69-9885-676f86520516\"},{\"content\":{\"connectorIds\":[],\"side\":\"TOP\"},\"type\":\"ConnectorPlacement.EquallySpacedRectSide\",\"uuid\":\"507b0a08-3f41-418e-b758-bf3c30bff976\"}]},\"type\":\"ConnectorPlacement.EquallySpacedConnector\",\"uuid\":\"3d035927-e5ab-4804-9878-aec4e1ed4314\"}],\"packageUris\":[\"http://schema.mathworks.com/mf0/Connector/R2020b\"],\"version\":\"1.0\"}"
  Projector : Subsystem  Description=Projector connected to a computer, capable of projecting on a smooth wall everything necessary to carry out the target test.
      settings: PortSchema="{\"entries\":[{\"content\":{\"headerSize\":26,\"margin\":15,\"minimumSpacing\":25,\"sides\":[{\"content\":{\"connectorIds\":[]},\"type\":\"ConnectorPlacement.EquallySpacedRectSide\",\"uuid\":\"036f86a6-46aa-44c7-aacf-5c5bf73f23a6\"},{\"content\":{\"connectorIds\":[\"Out1\"],\"side\":\"RIGHT\"},\"type\":\"ConnectorPlacement.EquallySpacedRectSide\",\"uuid\":\"14d10c07-b9d4-4e69-9885-676f86520516\"},{\"content\":{\"connectorIds\":[],\"side\":\"TOP\"},\"type\":\"ConnectorPlacement.EquallySpacedRectSide\",\"uuid\":\"507b0a08-3f41-418e-b758-bf3c30bff976\"}]},\"type\":\"ConnectorPlacement.EquallySpacedConnector\",\"uuid\":\"3d035927-e5ab-4804-9878-aec4e1ed4314\"}],\"packageUris\":[\"http://schema.mathworks.com/mf0/Connector/R2020b\"],\"version\":\"1.0\"}"
  Bus Element Out2 : Outport  PortName=Start
  Bus Element Out3 : Outport  Port=2  PortName=Lines
  Bus Element Out4 : Outport  Port=3  PortName=Proyection
  Bus Element Out1 : Outport  Port=4  PortName=obs
  wires:
  Obstacles/1(obs) -> Bus Element Out1/1
  Horn/1(Start) -> Bus Element Out2/1
  Insulating tapes/1(Lines) -> Bus Element Out3/1
  Projector/1(Proyection) -> Bus Element Out4/1

== system SystemComposerModel/Competition/Organization ==
  Before the competition : Subsystem
      settings: PortSchema="{\"entries\":[{\"content\":{\"headerSize\":26,\"margin\":15,\"minimumSpacing\":25,\"sides\":[{\"content\":{\"connectorIds\":[]},\"type\":\"ConnectorPlacement.EquallySpacedRectSide\",\"uuid\":\"d34c32ef-3d27-469b-8a35-abebe5333993\"},{\"content\":{\"connectorIds\":[],\"side\":\"RIGHT\"},\"type\":\"ConnectorPlacement.EquallySpacedRectSide\",\"uuid\":\"0a2917af-f234-4cdf-997c-680a118988b7\"},{\"content\":{\"connectorIds\":[],\"side\":\"TOP\"},\"type\":\"ConnectorPlacement.EquallySpacedRectSide\",\"uuid\":\"dcac7d54-9fff-4582-ba14-08bcbac36cd8\"}]},\"type\":\"ConnectorPlacement.EquallySpacedConnector\",\"uuid\":\"84591ee6-ffcc-49ff-97f7-997353b331d9\"}],\"packageUris\":[\"http://schema.mathworks.com/mf0/Connector/R2020b\"],\"version\":\"1.0\"}"
  During the competition : Subsystem
      settings: PortSchema="{\"entries\":[{\"content\":{\"headerSize\":26,\"margin\":15,\"minimumSpacing\":25,\"sides\":[{\"content\":{\"connectorIds\":[]},\"type\":\"ConnectorPlacement.EquallySpacedRectSide\",\"uuid\":\"d34c32ef-3d27-469b-8a35-abebe5333993\"},{\"content\":{\"connectorIds\":[],\"side\":\"RIGHT\"},\"type\":\"ConnectorPlacement.EquallySpacedRectSide\",\"uuid\":\"0a2917af-f234-4cdf-997c-680a118988b7\"},{\"content\":{\"connectorIds\":[],\"side\":\"TOP\"},\"type\":\"ConnectorPlacement.EquallySpacedRectSide\",\"uuid\":\"dcac7d54-9fff-4582-ba14-08bcbac36cd8\"}]},\"type\":\"ConnectorPlacement.EquallySpacedConnector\",\"uuid\":\"84591ee6-ffcc-49ff-97f7-997353b331d9\"}],\"packageUris\":[\"http://schema.mathworks.com/mf0/Connector/R2020b\"],\"version\":\"1.0\"}"

== system SystemComposerModel/Competition/People ==
  Audience : Subsystem
      settings: PortSchema="{\"entries\":[{\"content\":{\"headerSize\":26,\"margin\":15,\"minimumSpacing\":25,\"sides\":[{\"content\":{\"connectorIds\":[]},\"type\":\"ConnectorPlacement.EquallySpacedRectSide\",\"uuid\":\"036f86a6-46aa-44c7-aacf-5c5bf73f23a6\"},{\"content\":{\"connectorIds\":[],\"side\":\"RIGHT\"},\"type\":\"ConnectorPlacement.EquallySpacedRectSide\",\"uuid\":\"14d10c07-b9d4-4e69-9885-676f86520516\"},{\"content\":{\"connectorIds\":[],\"side\":\"TOP\"},\"type\":\"ConnectorPlacement.EquallySpacedRectSide\",\"uuid\":\"507b0a08-3f41-418e-b758-bf3c30bff976\"}]},\"type\":\"ConnectorPlacement.EquallySpacedConnector\",\"uuid\":\"3d035927-e5ab-4804-9878-aec4e1ed4314\"}],\"packageUris\":[\"http://schema.mathworks.com/mf0/Connector/R2020b\"],\"version\":\"1.0\"}"
  Observers : Subsystem
      settings: PortSchema="{\"entries\":[{\"content\":{\"headerSize\":26,\"margin\":15,\"minimumSpacing\":25,\"sides\":[{\"content\":{\"connectorIds\":[]},\"type\":\"ConnectorPlacement.EquallySpacedRectSide\",\"uuid\":\"036f86a6-46aa-44c7-aacf-5c5bf73f23a6\"},{\"content\":{\"connectorIds\":[],\"side\":\"RIGHT\"},\"type\":\"ConnectorPlacement.EquallySpacedRectSide\",\"uuid\":\"14d10c07-b9d4-4e69-9885-676f86520516\"},{\"content\":{\"connectorIds\":[],\"side\":\"TOP\"},\"type\":\"ConnectorPlacement.EquallySpacedRectSide\",\"uuid\":\"507b0a08-3f41-418e-b758-bf3c30bff976\"}]},\"type\":\"ConnectorPlacement.EquallySpacedConnector\",\"uuid\":\"3d035927-e5ab-4804-9878-aec4e1ed4314\"}],\"packageUris\":[\"http://schema.mathworks.com/mf0/Connector/R2020b\"],\"version\":\"1.0\"}"
  Participants : Subsystem
      settings: PortSchema="{\"entries\":[{\"content\":{\"headerSize\":26,\"margin\":15,\"minimumSpacing\":25,\"sides\":[{\"content\":{\"connectorIds\":[]},\"type\":\"ConnectorPlacement.EquallySpacedRectSide\",\"uuid\":\"036f86a6-46aa-44c7-aacf-5c5bf73f23a6\"},{\"content\":{\"connectorIds\":[],\"side\":\"RIGHT\"},\"type\":\"ConnectorPlacement.EquallySpacedRectSide\",\"uuid\":\"14d10c07-b9d4-4e69-9885-676f86520516\"},{\"content\":{\"connectorIds\":[],\"side\":\"TOP\"},\"type\":\"ConnectorPlacement.EquallySpacedRectSide\",\"uuid\":\"507b0a08-3f41-418e-b758-bf3c30bff976\"}]},\"type\":\"ConnectorPlacement.EquallySpacedConnector\",\"uuid\":\"3d035927-e5ab-4804-9878-aec4e1ed4314\"}],\"packageUris\":[\"http://schema.mathworks.com/mf0/Connector/R2020b\"],\"version\":\"1.0\"}"

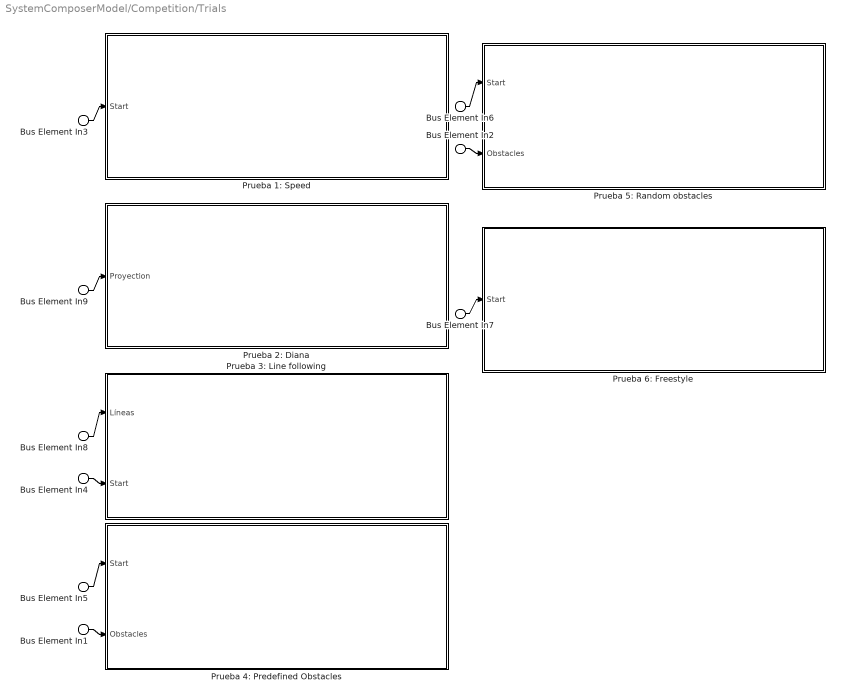
== system SystemComposerModel/Competition/Trials ==
  Bus Element In{3..7} (5 alike) : Inport  PortName=Start
  Bus Element In8 : Inport  Port=2  PortName=Lines
  Bus Element In9 : Inport  Port=3  PortName=Proyection
  Bus Element In1 : Inport  Port=4  PortName=Obs
  Bus Element In2 : Inport  Port=4  PortName=Obs
  Prueba 1: Speed : Subsystem
      settings: PortSchema="{\"entries\":[{\"content\":{\"headerSize\":26,\"margin\":15,\"minimumSpacing\":25,\"sides\":[{\"content\":{\"connectorIds\":[\"In1\"]},\"type\":\"ConnectorPlacement.EquallySpacedRectSide\",\"uuid\":\"036f86a6-46aa-44c7-aacf-5c5bf73f23a6\"},{\"content\":{\"connectorIds\":[],\"side\":\"RIGHT\"},\"type\":\"ConnectorPlacement.EquallySpacedRectSide\",\"uuid\":\"14d10c07-b9d4-4e69-9885-676f86520516\"},{\"content\":{\"connectorIds\":[],\"side\":\"TOP\"},\"type\":\"ConnectorPlacement.EquallySpacedRectSide\",\"uuid\":\"507b0a08-3f41-418e-b758-bf3c30bff976\"}]},\"type\":\"ConnectorPlacement.EquallySpacedConnector\",\"uuid\":\"3d035927-e5ab-4804-9878-aec4e1ed4314\"}],\"packageUris\":[\"http://schema.mathworks.com/mf0/Connector/R2020b\"],\"version\":\"1.0\"}"
  Prueba 2: Diana : Subsystem
      settings: PortSchema="{\"entries\":[{\"content\":{\"headerSize\":26,\"margin\":15,\"minimumSpacing\":25,\"sides\":[{\"content\":{\"connectorIds\":[\"In1\"]},\"type\":\"ConnectorPlacement.EquallySpacedRectSide\",\"uuid\":\"036f86a6-46aa-44c7-aacf-5c5bf73f23a6\"},{\"content\":{\"connectorIds\":[],\"side\":\"RIGHT\"},\"type\":\"ConnectorPlacement.EquallySpacedRectSide\",\"uuid\":\"14d10c07-b9d4-4e69-9885-676f86520516\"},{\"content\":{\"connectorIds\":[],\"side\":\"TOP\"},\"type\":\"ConnectorPlacement.EquallySpacedRectSide\",\"uuid\":\"507b0a08-3f41-418e-b758-bf3c30bff976\"}]},\"type\":\"ConnectorPlacement.EquallySpacedConnector\",\"uuid\":\"3d035927-e5ab-4804-9878-aec4e1ed4314\"}],\"packageUris\":[\"http://schema.mathworks.com/mf0/Connector/R2020b\"],\"version\":\"1.0\"}"
  Prueba 3: Line following : Subsystem
      settings: PortSchema="{\"entries\":[{\"content\":{\"headerSize\":26,\"margin\":15,\"minimumSpacing\":25,\"sides\":[{\"content\":{\"connectorIds\":[\"In1\",\"In2\"]},\"type\":\"ConnectorPlacement.EquallySpacedRectSide\",\"uuid\":\"036f86a6-46aa-44c7-aacf-5c5bf73f23a6\"},{\"content\":{\"connectorIds\":[],\"side\":\"RIGHT\"},\"type\":\"ConnectorPlacement.EquallySpacedRectSide\",\"uuid\":\"14d10c07-b9d4-4e69-9885-676f86520516\"},{\"content\":{\"connectorIds\":[],\"side\":\"TOP\"},\"type\":\"ConnectorPlacement.EquallySpacedRectSide\",\"uuid\":\"507b0a08-3f41-418e-b758-bf3c30bff976\"}]},\"type\":\"ConnectorPlacement.EquallySpacedConnector\",\"uuid\":\"3d035927-e5ab-4804-9878-aec4e1ed4314\"}],\"packageUris\":[\"http://schema.mathworks.com/mf0/Connector/R2020b\"],\"version\":\"1.0\"}"
  Prueba 4: Predefined Obstacles : Subsystem
      settings: PortSchema="{\"entries\":[{\"content\":{\"headerSize\":26,\"margin\":15,\"minimumSpacing\":25,\"sides\":[{\"content\":{\"connectorIds\":[\"In1\",\"In2\"]},\"type\":\"ConnectorPlacement.EquallySpacedRectSide\",\"uuid\":\"036f86a6-46aa-44c7-aacf-5c5bf73f23a6\"},{\"content\":{\"connectorIds\":[],\"side\":\"RIGHT\"},\"type\":\"ConnectorPlacement.EquallySpacedRectSide\",\"uuid\":\"14d10c07-b9d4-4e69-9885-676f86520516\"},{\"content\":{\"connectorIds\":[],\"side\":\"TOP\"},\"type\":\"ConnectorPlacement.EquallySpacedRectSide\",\"uuid\":\"507b0a08-3f41-418e-b758-bf3c30bff976\"}]},\"type\":\"ConnectorPlacement.EquallySpacedConnector\",\"uuid\":\"3d035927-e5ab-4804-9878-aec4e1ed4314\"}],\"packageUris\":[\"http://schema.mathworks.com/mf0/Connector/R2020b\"],\"version\":\"1.0\"}"
  Prueba 5: Random obstacles : Subsystem
      settings: PortSchema="{\"entries\":[{\"content\":{\"headerSize\":26,\"margin\":15,\"minimumSpacing\":25,\"sides\":[{\"content\":{\"connectorIds\":[\"In1\",\"In2\"]},\"type\":\"ConnectorPlacement.EquallySpacedRectSide\",\"uuid\":\"036f86a6-46aa-44c7-aacf-5c5bf73f23a6\"},{\"content\":{\"connectorIds\":[],\"side\":\"RIGHT\"},\"type\":\"ConnectorPlacement.EquallySpacedRectSide\",\"uuid\":\"14d10c07-b9d4-4e69-9885-676f86520516\"},{\"content\":{\"connectorIds\":[],\"side\":\"TOP\"},\"type\":\"ConnectorPlacement.EquallySpacedRectSide\",\"uuid\":\"507b0a08-3f41-418e-b758-bf3c30bff976\"}]},\"type\":\"ConnectorPlacement.EquallySpacedConnector\",\"uuid\":\"3d035927-e5ab-4804-9878-aec4e1ed4314\"}],\"packageUris\":[\"http://schema.mathworks.com/mf0/Connector/R2020b\"],\"version\":\"1.0\"}"
  Prueba 6: Freestyle : Subsystem
      settings: PortSchema="{\"entries\":[{\"content\":{\"headerSize\":26,\"margin\":15,\"minimumSpacing\":25,\"sides\":[{\"content\":{\"connectorIds\":[\"In1\"]},\"type\":\"ConnectorPlacement.EquallySpacedRectSide\",\"uuid\":\"036f86a6-46aa-44c7-aacf-5c5bf73f23a6\"},{\"content\":{\"connectorIds\":[],\"side\":\"RIGHT\"},\"type\":\"ConnectorPlacement.EquallySpacedRectSide\",\"uuid\":\"14d10c07-b9d4-4e69-9885-676f86520516\"},{\"content\":{\"connectorIds\":[],\"side\":\"TOP\"},\"type\":\"ConnectorPlacement.EquallySpacedRectSide\",\"uuid\":\"507b0a08-3f41-418e-b758-bf3c30bff976\"}]},\"type\":\"ConnectorPlacement.EquallySpacedConnector\",\"uuid\":\"3d035927-e5ab-4804-9878-aec4e1ed4314\"}],\"packageUris\":[\"http://schema.mathworks.com/mf0/Connector/R2020b\"],\"version\":\"1.0\"}"
  wires:
  Bus Element In1/1 -> Prueba 4: Predefined Obstacles/2(Obstacles)
  Bus Element In2/1 -> Prueba 5: Random obstacles/2(Obstacles)
  Bus Element In3/1 -> Prueba 1: Speed/1(Start)
  Bus Element In4/1 -> Prueba 3: Line following/2(Start)
  Bus Element In5/1 -> Prueba 4: Predefined Obstacles/1(Start)
  Bus Element In6/1 -> Prueba 5: Random obstacles/1(Start)
  Bus Element In7/1 -> Prueba 6: Freestyle/1(Start)
  Bus Element In8/1 -> Prueba 3: Line following/1(Líneas)
  Bus Element In9/1 -> Prueba 2: Diana/1(Proyection)

== system SystemComposerModel/Crazyflie 2.0/Camara ==
  Bus Element Out1 : Outport  PortName=VideoBus

== system SystemComposerModel/Crazyflie 2.0/ClimConditions ==
  Bus Element In1 : Inport  PortName=Enviroment
  Wind : Subsystem
      settings: PortSchema="{\"entries\":[{\"content\":{\"headerSize\":26,\"margin\":15,\"minimumSpacing\":25,\"sides\":[{\"content\":{\"connectorIds\":[\"In1\"]},\"type\":\"ConnectorPlacement.EquallySpacedRectSide\",\"uuid\":\"b8d7d09c-e9ae-43de-8d46-f99ec2351e24\"},{\"content\":{\"connectorIds\":[\"Out1\",\"Out2\",\"Out3\"],\"side\":\"RIGHT\"},\"type\":\"ConnectorPlacement.EquallySpacedRectSide\",\"uuid\":\"4693648e-b0a2-4db8-a983-4bee2f51d894\"},{\"content\":{\"connectorIds\":[],\"side\":\"TOP\"},\"type\":\"ConnectorPlacement.EquallySpacedRectSide\",\"uuid\":\"9f0e5fe3-4fa7-4597-a4df-94b2d5032736\"}]},\"type\":\"ConnectorPlacement.EquallySpacedConnector\",\"uuid\":\"297bf07a-4341-4423-8aed-0af6edbe7857\"}],\"packageUris\":[\"http://schema.mathworks.com/mf0/Connector/R2020b\"],\"version\":\"1.0\"}"
  Bus Element Out1 : Outport  PortName=F_x_in
  Bus Element Out2 : Outport  Port=2  PortName=F_y_in
  Bus Element Out3 : Outport  Port=3  PortName=F_z_in
  wires:
  Bus Element In1/1 -> Wind/1(Enviroment)
  Wind/1(F_x_in) -> Bus Element Out1/1
  Wind/2(F_y_in) -> Bus Element Out2/1
  Wind/3(F_z_in) -> Bus Element Out3/1

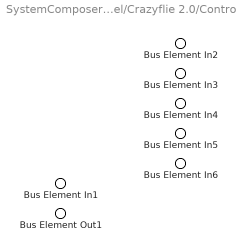
== system SystemComposerModel/Crazyflie 2.0/Controller ==
  Bus Element In2 : Inport  PortName=Reference
  Bus Element In6 : Inport  Port=2  PortName=CodeModifications
  Bus Element In3 : Inport  Port=3  PortName=F_x_in
  Bus Element In4 : Inport  Port=4  PortName=F_y_in
  Bus Element In5 : Inport  Port=5  PortName=F_z_in
  Bus Element In1 : Inport  Port=6  PortName=Estimated State
  Bus Element Out1 : Outport  PortName=Actuation Signal

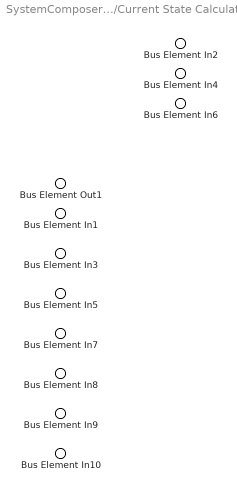
== system SystemComposerModel/Crazyflie 2.0/Current State Calculation ==
  Bus Element In6 : Inport  PortName=d_roll
  Bus Element In2 : Inport  Port=2  PortName=dist_rear
  Bus Element In1 : Inport  Port=3  PortName=dist_front
  Bus Element In4 : Inport  Port=4  PortName=dist_left
  Bus Element In3 : Inport  Port=5  PortName=dist_right
  Bus Element In5 : Inport  Port=6  PortName=d_pitch
  Bus Element In7 : Inport  Port=7  PortName=d_yaw
  Bus Element In8 : Inport  Port=8  PortName=acc_x
  Bus Element In9 : Inport  Port=9  PortName=acc_y
  Bus Element In10 : Inport  Port=10  PortName=acc_z
  Bus Element Out1 : Outport  PortName=Current State

== system SystemComposerModel/Crazyflie 2.0/Functional-Logic ==
  Bus Element In1 : Inport  PortName=GCSCmds

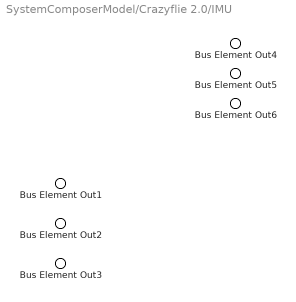
== system SystemComposerModel/Crazyflie 2.0/IMU ==
  Bus Element Out5 : Outport  PortName=d_pitch
  Bus Element Out6 : Outport  Port=2  PortName=d_roll
  Bus Element Out4 : Outport  Port=3  PortName=d_yaw
  Bus Element Out1 : Outport  Port=4  PortName=acc_x
  Bus Element Out2 : Outport  Port=5  PortName=acc_y
  Bus Element Out3 : Outport  Port=6  PortName=acc_z

== system SystemComposerModel/Crazyflie 2.0/Motor 1 ==
  Bus Element In1 : Inport  PortName=Motor1_PWM

== system SystemComposerModel/Crazyflie 2.0/Motor 2 ==
  Bus Element In1 : Inport  PortName=Motor2_PWM

== system SystemComposerModel/Crazyflie 2.0/Motor 3 ==
  Bus Element In1 : Inport  PortName=Motor3_PWM

== system SystemComposerModel/Crazyflie 2.0/Motor 4 ==
  Bus Element In1 : Inport  PortName=Motor4_PWM

== system SystemComposerModel/Crazyflie 2.0/PWM Generator ==
  Bus Element In1 : Inport  PortName=Actuation Signal
  Bus Element Out1 : Outport  PortName=Motor1_PWM
  Bus Element Out2 : Outport  Port=2  PortName=Motor2_PWM
  Bus Element Out3 : Outport  Port=3  PortName=Motor3_PWM
  Bus Element Out4 : Outport  Port=4  PortName=Motor4_PWM
